simulink model "VCU_M1"  (R2026a)
settings: Solver=FixedStepDiscrete  StopTime=inf  FixedStep=0.0005  EnableMultiTasking=on
libraries: stm32blockslib x5
settings Model: STM32="{\"CANWrite\":{\"ID\":\"3\"},\"UARTWrite\":{\"ID\":\"4\"},\"CANRead\":{\"ID\":\"5\"},\"AnalogInput\":{\"ID\":\"1\"},\"DigitalPortWrite\":{\"ID\":\"8\"}}"  Creator=1011472417  LastModifiedBy=1011472417
settings HardwareCC: ProdLargestAtomicInteger=Long  ProdLargestAtomicFloat=Double  ProdHWDeviceType=ARM Compatible->ARM Cortex-M
settings RTWCC: SystemTargetFile=ert.tlc  HardwareBoard=STM32F1xx Based  TLCOptions=-aInlineSetEventsForThisBaseRateFcn=TLC_FALSE -aSuppressMultiTaskScheduler=TLC_FALSE -aRateBasedStepFcn=1  Toolchain=GNU Tools for STM32  BuildConfiguration=Faster Runs  Description=Embedded Coder
settings ERTTargetCC: ExtModeTransport=3.0  ExtModeStaticAllocSize=2048.0  CodeReplacementLibrary=ARM Cortex-M

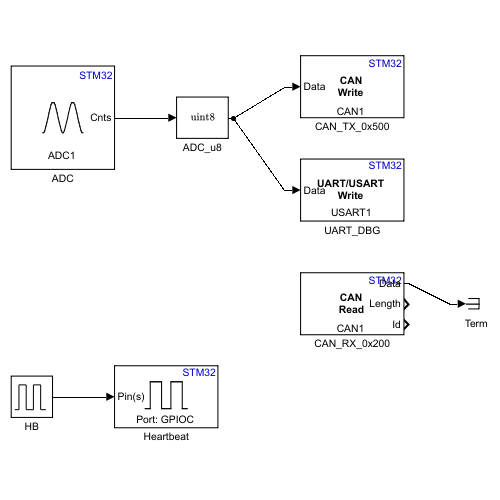
[thumbnail: Simulink's stored preview of the top-level diagram]
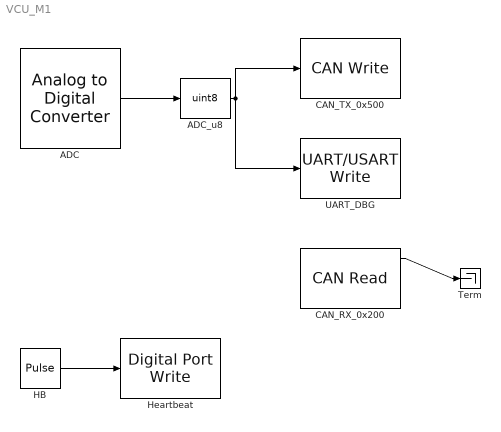
== system VCU_M1 ==
  ADC : stm32blockslib/Analog to Digital Converter  ADCModule=ADC1  ConversionGroup=Regular  TriggerMode=Trigger and read  NumberOfConversions=8  EnableBufferConv=off  BufferLength=1  OutputStatus=off  SampleTime=-1
  ADC_u8 : DataTypeConversion  OutDataTypeStr=uint8  SaturateOnIntegerOverflow=off  RndMeth=Floor
  CAN_RX_0x200 : stm32blockslib/CAN Read  CANModule=CAN1  BlockMode=Receive  OperationReadMode=Data  OperationWriteMode=Data  OutputTypeReadMode=Unpacked  DataFormatWriteMode=Raw data  ReadSource=FIFO 0  IdentifierTypeVia=Dialog  IdentifierType=Standard (11-bit identifier)  IdentifierVia=Inport  Identifier=100  DataLengthVia=Inport  DataLength=8  OutputIdType=off  TransmitRemoteFrame=off  OutputRemoteFrame=off  OutputTxFifoLevel=off  OutputRxFifoLevel=off  OutputStatus=off  Timeout=0.001  SampleTime=-1
  CAN_TX_0x500 : stm32blockslib/CAN Write  CANModule=CAN1  BlockMode=Transmit  OperationReadMode=Data  OperationWriteMode=Data  OutputTypeReadMode=Unpacked  DataFormatWriteMode=Raw data  ReadSource=FIFO 0  IdentifierTypeVia=Dialog  IdentifierType=Standard (11-bit identifier)  IdentifierVia=Dialog  Identifier=1280  DataLengthVia=Dialog  DataLength=8  OutputIdType=off  TransmitRemoteFrame=off  OutputRemoteFrame=off  OutputTxFifoLevel=off  OutputRxFifoLevel=off  OutputStatus=off  Timeout=0.001  SampleTime=-1
  HB : DiscretePulseGenerator  PulseType=Time based  PulseWidth=50  SampleTime=0.0005
  Heartbeat : stm32blockslib/Digital Port Write  PortName=GPIOC  PinNumber=[13]  ReadOperation=off  IOAsArray=on  SampleTime=-1
  Term : Terminator
  UART_DBG : stm32blockslib/UART//USART Write  UARTModule=USART1  LengthOfDataToSend=off  BlockingMode=off  BlockingTimeout=0.1  OutputStatus=off
  wires:
  ADC/1 -> ADC_u8/1
  ADC_u8/1 -> CAN_TX_0x500/1, UART_DBG/1
  CAN_RX_0x200/1 -> Term/1
  HB/1 -> Heartbeat/1
